simulink model "Roadsense_SafetySupervisor"  (R2025b)
settings: Solver=FixedStepDiscrete  StartTime=0.0  StopTime=1.0  FixedStep=RsTsBase  RelTol=1e-3
undefined symbols (not defined in the file or in its folder): RsGridCols, RsGridRows, RsMaxTracks, RsSafetyEmergencyHoldTicks, RsSafetyRecoveryTicks, RsTsControl
settings Model: DataDictionary=Roadsense_Data.sldd  Creator=ragur  LastModifiedBy=ragur

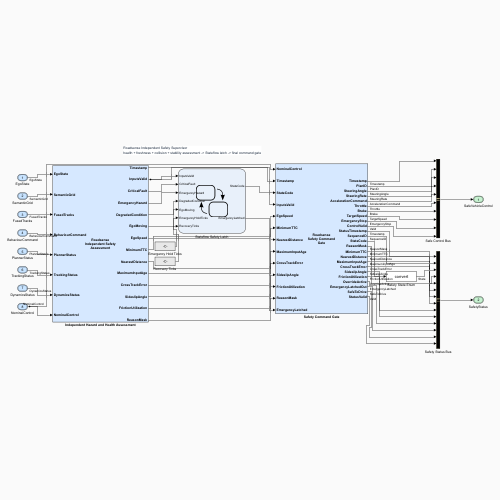
[thumbnail: Simulink's stored preview of the top-level diagram]
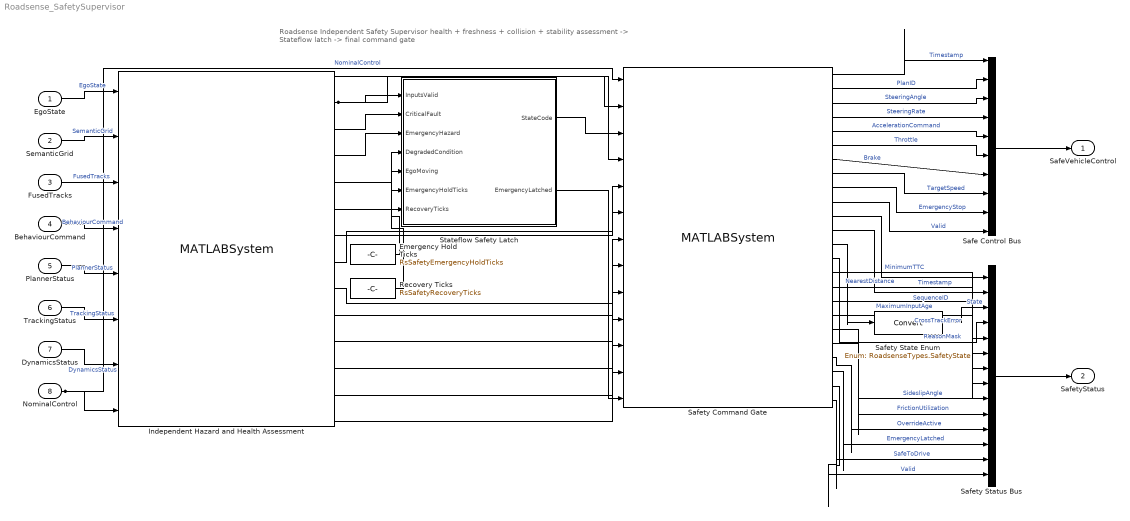
== system Roadsense_SafetySupervisor ==
  note: Roadsense Independent Safety Supervisor
      | health + freshness + collision + stability assessment -> Stateflow latch -> final command gate
  EgoState : Inport  OutDataTypeStr=Bus: RsEgoStateBus  PortDimensions=1  SampleTime=RsTsControl
  SemanticGrid : Inport  Port=2  OutDataTypeStr=Bus: RsSemanticGridBus  PortDimensions=1  SampleTime=RsTsControl
  FusedTracks : Inport  Port=3  OutDataTypeStr=Bus: RsFusedTrackListBus  PortDimensions=1  SampleTime=RsTsControl
  BehaviourCommand : Inport  Port=4  OutDataTypeStr=Bus: RsBehaviourCommandBus  PortDimensions=1  SampleTime=RsTsControl
  PlannerStatus : Inport  Port=5  OutDataTypeStr=Bus: RsPlannerStatusBus  PortDimensions=1  SampleTime=RsTsControl
  TrackingStatus : Inport  Port=6  OutDataTypeStr=Bus: RsTrackingStatusBus  PortDimensions=1  SampleTime=RsTsControl
  DynamicsStatus : Inport  Port=7  OutDataTypeStr=Bus: RsVehicleDynamicsStatusBus  PortDimensions=1  SampleTime=RsTsControl
  NominalControl : Inport  Port=8  OutDataTypeStr=Bus: RsVehicleControlBus  PortDimensions=1  SampleTime=RsTsControl
  Emergency Hold Ticks : Constant  Value=RsSafetyEmergencyHoldTicks  OutDataTypeStr=uint16
  Independent Hazard and Health Assessment : MATLABSystem  System=RoadsenseSafetyAssessmentSystem  MaxTracks=double(RsMaxTracks)  GridRows=double(RsGridRows)  GridCols=double(RsGridCols)  GridResolution=RsGridResolution  GridXLimits=RsGridXLimits  GridYLimits=RsGridYLimits  EmergencyTTC=RsSafetyEmergencyTTC  EmergencyDistance=RsSafetyEmergencyDistance  ControlStaleTime=RsSafetyControlStaleTime  TrackingStaleTime=RsSafetyTrackingStaleTime  PerceptionStaleTime=RsSafetyPerceptionStaleTime  PlanningStaleTime=RsSafetyPlanningStaleTime  CrossTrackWarning=RsSafetyCrossTrackWarning  CrossTrackFault=RsSafetyCrossTrackFault  HeadingWarning=RsSafetyHeadingWarning  HeadingFault=RsSafetyHeadingFault  SideslipWarning=RsSafetySideslipWarning  SideslipFault=RsSafetySideslipFault  FrictionWarning=RsSafetyFrictionWarning  LateralAccelerationFault=RsSafetyLateralAccelerationFault  SimulateUsing=Code generation
      mask Type: RoadsenseSafetyAssessmentSystem
  Recovery Ticks : Constant  Value=RsSafetyRecoveryTicks  OutDataTypeStr=uint16
  Safe Control Bus : BusCreator  Inputs=10  OutDataTypeStr=Bus: RsVehicleControlBus
  Safety Command Gate : MATLABSystem  System=RoadsenseSafetyCommandSystem  MaximumSteering=RsControllerMaximumSteering  EmergencyDeceleration=RsBehaviourEmergencyDeceleration  MinimalRiskDeceleration=RsSafetyMinimalRiskDeceleration  DegradedSpeed=RsSafetyDegradedSpeed  SimulateUsing=Code generation
      mask Type: RoadsenseSafetyCommandSystem
  Safety State Enum : DataTypeConversion  OutDataTypeStr=Enum: RoadsenseTypes.SafetyState  SaturateOnIntegerOverflow=off  RndMeth=Floor
  Safety Status Bus : BusCreator  Inputs=14  OutDataTypeStr=Bus: RsSafetyStatusBus
  Stateflow Safety Latch : Stateflow chart  TreatAsAtomicUnit=on
  SafeVehicleControl : Outport  OutDataTypeStr=Bus: RsVehicleControlBus
  SafetyStatus : Outport  Port=2  OutDataTypeStr=Bus: RsSafetyStatusBus
  wires:
  EgoState/1 -> Independent Hazard and Health Assessment/1  "EgoState"
  SemanticGrid/1 -> Independent Hazard and Health Assessment/2  "SemanticGrid"
  FusedTracks/1 -> Independent Hazard and Health Assessment/3  "FusedTracks"
  BehaviourCommand/1 -> Independent Hazard and Health Assessment/4  "BehaviourCommand"
  PlannerStatus/1 -> Independent Hazard and Health Assessment/5  "PlannerStatus"
  TrackingStatus/1 -> Independent Hazard and Health Assessment/6  "TrackingStatus"
  DynamicsStatus/1 -> Independent Hazard and Health Assessment/7  "DynamicsStatus"
  NominalControl/1 -> Independent Hazard and Health Assessment/8, Safety Command Gate/1  "NominalControl"
  Independent Hazard and Health Assessment/2 -> Stateflow Safety Latch/1(InputsValid), Safety Command Gate/4
  Independent Hazard and Health Assessment/3 -> Stateflow Safety Latch/2(CriticalFault)
  Independent Hazard and Health Assessment/4 -> Stateflow Safety Latch/3(EmergencyHazard)
  Independent Hazard and Health Assessment/5 -> Stateflow Safety Latch/4(DegradedCondition)
  Independent Hazard and Health Assessment/6 -> Stateflow Safety Latch/5(EgoMoving)
  Emergency Hold Ticks/1 -> Stateflow Safety Latch/6(EmergencyHoldTicks)
  Recovery Ticks/1 -> Stateflow Safety Latch/7(RecoveryTicks)
  Independent Hazard and Health Assessment/1 -> Safety Command Gate/2
  Stateflow Safety Latch/1(StateCode) -> Safety Command Gate/3
  Independent Hazard and Health Assessment/7 -> Safety Command Gate/5
  Independent Hazard and Health Assessment/8 -> Safety Command Gate/6
  Independent Hazard and Health Assessment/9 -> Safety Command Gate/7
  Independent Hazard and Health Assessment/10 -> Safety Command Gate/8
  Independent Hazard and Health Assessment/11 -> Safety Command Gate/9
  Independent Hazard and Health Assessment/12 -> Safety Command Gate/10
  Independent Hazard and Health Assessment/13 -> Safety Command Gate/11
  Independent Hazard and Health Assessment/14 -> Safety Command Gate/12
  Stateflow Safety Latch/2(EmergencyLatched) -> Safety Command Gate/13
  Safety Command Gate/13 -> Safety State Enum/1
  Safety Command Gate/1 -> Safe Control Bus/1  "Timestamp"
  Safety Command Gate/2 -> Safe Control Bus/2  "PlanID"
  Safety Command Gate/3 -> Safe Control Bus/3  "SteeringAngle"
  Safety Command Gate/4 -> Safe Control Bus/4  "SteeringRate"
  Safety Command Gate/5 -> Safe Control Bus/5  "AccelerationCommand"
  Safety Command Gate/6 -> Safe Control Bus/6  "Throttle"
  Safety Command Gate/7 -> Safe Control Bus/7  "Brake"
  Safety Command Gate/8 -> Safe Control Bus/8  "TargetSpeed"
  Safety Command Gate/9 -> Safe Control Bus/9  "EmergencyStop"
  Safety Command Gate/10 -> Safe Control Bus/10  "Valid"
  Safety Command Gate/11 -> Safety Status Bus/1  "Timestamp"
  Safety Command Gate/12 -> Safety Status Bus/2  "SequenceID"
  Safety State Enum/1 -> Safety Status Bus/3  "State"
  Safety Command Gate/14 -> Safety Status Bus/4  "ReasonMask"
  Safety Command Gate/15 -> Safety Status Bus/5  "MinimumTTC"
  Safety Command Gate/16 -> Safety Status Bus/6  "NearestDistance"
  Safety Command Gate/17 -> Safety Status Bus/7  "MaximumInputAge"
  Safety Command Gate/18 -> Safety Status Bus/8  "CrossTrackError"
  Safety Command Gate/19 -> Safety Status Bus/9  "SideslipAngle"
  Safety Command Gate/20 -> Safety Status Bus/10  "FrictionUtilization"
  Safety Command Gate/21 -> Safety Status Bus/11  "OverrideActive"
  Safety Command Gate/22 -> Safety Status Bus/12  "EmergencyLatched"
  Safety Command Gate/23 -> Safety Status Bus/13  "SafeToDrive"
  Safety Command Gate/24 -> Safety Status Bus/14  "Valid"
  Safe Control Bus/1 -> SafeVehicleControl/1
  Safety Status Bus/1 -> SafetyStatus/1

== stateflow chart Roadsense_SafetySupervisor/Stateflow Safety Latch ==
  state SafetyDecision
    entry:
    PreviousState = uint8(0);
    EmergencyCounter = uint16(0);
    RecoveryCounter = uint16(0);
    StateCode = uint8(0);
    EmergencyLatched = false;
    during:
    [StateCode, EmergencyCounter, RecoveryCounter, EmergencyLatched] = ...
    RoadsenseSafetyDecisionCore(InputsValid, CriticalFault, EmergencyHazard, ...
    DegradedCondition, EgoMoving, PreviousState, EmergencyCounter, ...
    RecoveryCounter, EmergencyHoldTicks, RecoveryTicks);
    PreviousState = StateCode;
  (default) -> SafetyDecision
  data: InputsValid input boolean; CriticalFault input boolean; EmergencyHazard input boolean; DegradedCondition input boolean; EgoMoving input boolean; EmergencyHoldTicks input uint16; RecoveryTicks input uint16; StateCode output uint8; EmergencyLatched output boolean; PreviousState local uint8; EmergencyCounter local uint16; RecoveryCounter local uint16
